simulink model "Model"  (R2020a)
settings: Solver=ode4  StartTime=0.0  StopTime=100  FixedStep=0.0005  RelTol=1e-3  EnableMultiTasking=on
libraries: simulink x2
settings Model: Creator=Cason  LastModifiedBy=Cason
settings OptimizationCC: BlockReduction=off  DefaultParameterBehavior=Inlined  BufferReuse=off

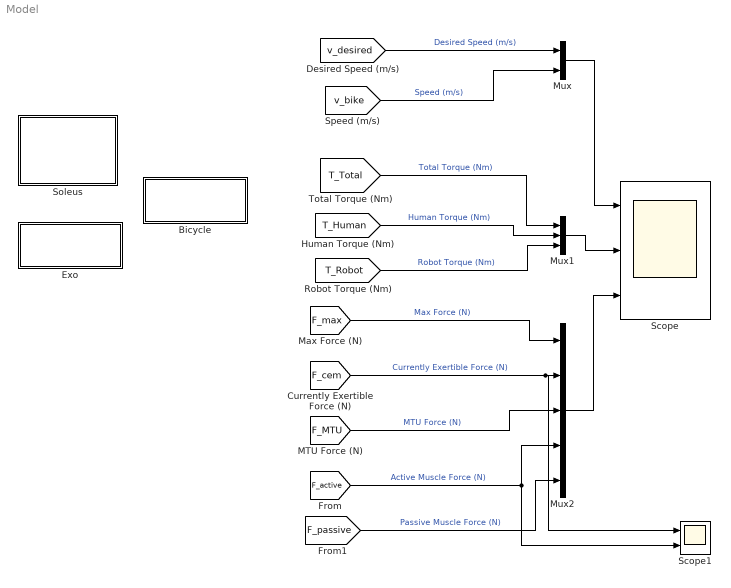
== system Model ==
  Bicycle : Subsystem
  Exo : Subsystem
  Mux : Mux  Inputs=2
  Mux1 : Mux  Inputs=3
  Mux2 : Mux  Inputs=5
  Scope : Scope  NumInputPorts=3
  Scope1 : Scope  NumInputPorts=2
  Soleus : Subsystem
  wires:
  Mux/1 -> Scope/1
  [v_desired] -> Mux/1  "Desired Speed (m/s)"
  [v_bike] -> Mux/2  "Speed (m/s)"
  Mux1/1 -> Scope/2
  [T_Human] -> Mux1/2  "Human Torque (Nm)"
  [T_Robot] -> Mux1/3  "Robot Torque (Nm)"
  [T_Total] -> Mux1/1  "Total Torque (Nm)"
  [F_max] -> Mux2/1  "Max Force (N)"
  [F_cem] -> Scope1/1, Mux2/2  "Currently Exertible Force (N)"
  [F_MTU] -> Mux2/3  "MTU Force (N)"
  Mux2/1 -> Scope/3
  [F_active] -> Scope1/2, Mux2/4  "Active Muscle Force (N)"
  [F_passive] -> Mux2/5  "Passive Muscle Force (N)"

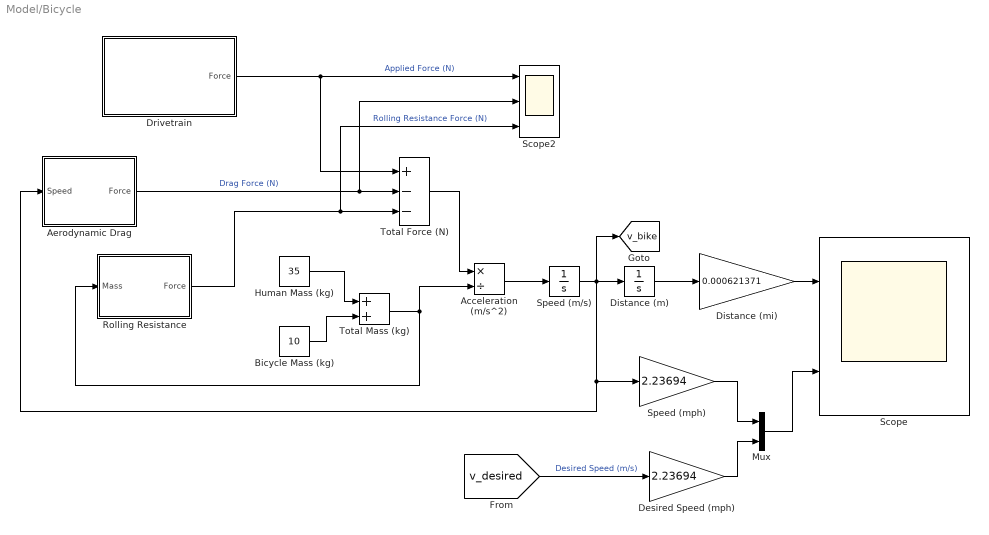
== system Model/Bicycle ==
  Acceleration (m/s^2) : Product  Inputs=*/
  Aerodynamic Drag : Subsystem
  Bicycle Mass (kg) : Constant  Value=10
  Desired Speed (mph) : Gain  Gain=2.23694
  Distance (m) : Integrator
  Distance (mi) : Gain  Gain=0.000621371
  Drivetrain : Subsystem
  Human Mass (kg) : Constant  Value=35
  Mux : Mux  Inputs=2
  Rolling Resistance : Subsystem
  Scope : Scope  NumInputPorts=2
  Scope2 : Scope  NumInputPorts=3
  Speed (m/s) : Integrator
  Speed (mph) : Gain  Gain=2.23694
  Total Force (N) : Sum  Inputs=+--
  Total Mass (kg) : Sum
  tag scope: v_bike=global
  wires:
  Human Mass (kg)/1 -> Total Mass (kg)/1
  Bicycle Mass (kg)/1 -> Total Mass (kg)/2
  Total Mass (kg)/1 -> Acceleration (m/s^2)/2, Rolling Resistance/1(Mass)
  Acceleration (m/s^2)/1 -> Speed (m/s)/1
  Speed (m/s)/1 -> [v_bike], Aerodynamic Drag/1(Speed), Speed (mph)/1, Distance (m)/1
  Distance (m)/1 -> Distance (mi)/1
  Total Force (N)/1 -> Acceleration (m/s^2)/1
  Rolling Resistance/1(Force) -> Total Force (N)/3, Scope2/3  "Rolling Resistance Force (N)"
  Aerodynamic Drag/1(Force) -> Scope2/2, Total Force (N)/2  "Drag Force (N)"
  Drivetrain/1(Force) -> Scope2/1, Total Force (N)/1  "Applied Force (N)"
  Distance (mi)/1 -> Scope/1
  Speed (mph)/1 -> Mux/1
  Mux/1 -> Scope/2
  [v_desired] -> Desired Speed (mph)/1  "Desired Speed (m/s)"
  Desired Speed (mph)/1 -> Mux/2

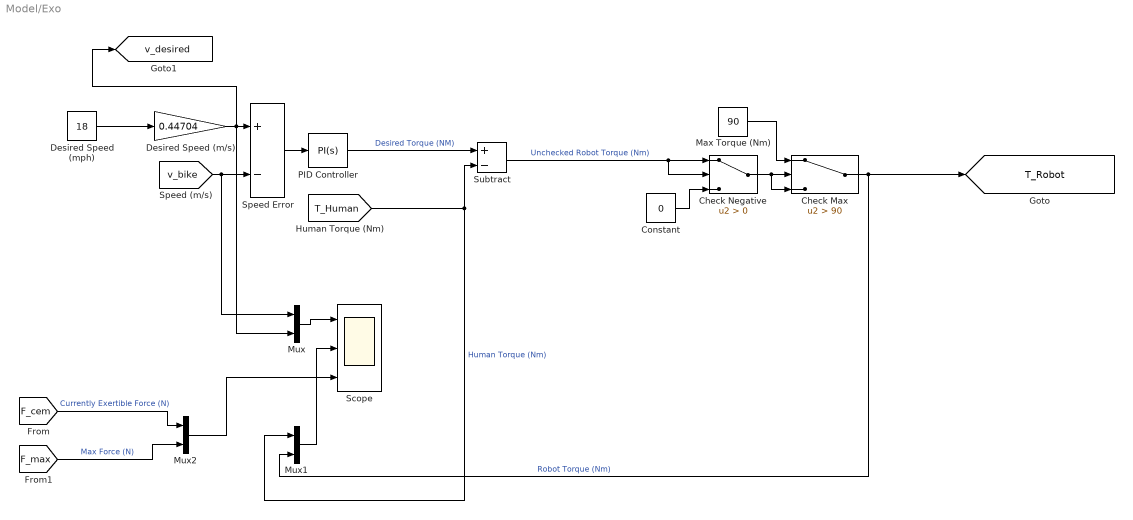
== system Model/Exo ==
  Check Max : Switch  Criteria=u2 > Threshold  Threshold=90
  Check Negative : Switch  Criteria=u2 > Threshold
  Constant : Constant  Value=0
  Desired Speed (m/s) : Gain  Gain=0.44704
  Desired Speed (mph) : Constant  Value=18
  Max Torque (Nm) : Constant  Value=90
  Mux : Mux  Inputs=2
  Mux1 : Mux  Inputs=2
  Mux2 : Mux  Inputs=2
  PID Controller : simulink/Continuous/PID Controller  Controller=PI  Form=Parallel  TimeDomain=Continuous-time  UseExternalTs=off  SampleTime=-1  IntegratorMethod=Forward Euler  FilterMethod=Forward Euler  ControllerParametersSource=internal  P=5  I=0.9  D=0.1  UseFilter=on  N=100  TunerSelectOption=Transfer Function Based (PID Tuner App)  InitialConditionSource=internal  InitialConditionForIntegrator=0  InitialConditionForFilter=0  DifferentiatorICPrevScaledInput=0  ExternalReset=none  TrackingMode=off  Kt=1  LimitOutput=off  UpperSaturationLimit=inf  LowerSaturationLimit=-inf  LinearizeAsGain=on  AntiWindupMode=none  Kb=1  POutMin=[]  POutMax=[]  IOutMin=[]  IOutMax=[]  DOutMin=[]  DOutMax=[]  NOutMin=[]  NOutMax=[]  SumOutMin=[]  SumOutMax=[]  SaturationOutMin=[]  SaturationOutMax=[]  PParamMin=[]  PParamMax=[]  IParamMin=[]  IParamMax=[]  DParamMin=[]  DParamMax=[]  NParamMin=[]  NParamMax=[]  KbParamMin=[]  KbParamMax=[]  KtParamMin=[]  KtParamMax=[]  KbOutMin=[]  KbOutMax=[]  KtOutMin=[]  KtOutMax=[]  IntegratorOutMin=[]  IntegratorOutMax=[]  FilterOutMin=[]  FilterOutMax=[]  SumI1OutMin=[]  SumI1OutMax=[]  SumI2OutMin=[]  SumI2OutMax=[]  SumI3OutMin=[]  SumI3OutMax=[]  SumI4OutMin=[]  SumI4OutMax=[]  SumDOutMin=[]  SumDOutMax=[]  DifferentiatorOutMin=[]  DifferentiatorOutMax=[]  FilterDiffOutCoefMin=[]  FilterDiffOutCoefMax=[]  ReciprocalOutMin=[]  ReciprocalOutMax=[]  SumDenOutMin=[]  SumDenOutMax=[]  SumNumOutMin=[]  SumNumOutMax=[]  DivideOutMin=[]  DivideOutMax=[]  UdiffTsProdOutMin=[]  UdiffTsProdOutMax=[]  NTsProdOutMin=[]  NTsProdOutMax=[]  UintegralTsProdOutMin=[]  UintegralTsProdOutMax=[]  UngainTsProdOutMin=[]  UngainTsProdOutMax=[]  IntegratorContinuousStateAttributes=''  IntegratorStateMustResolveToSignalObject=off  IntegratorRTWStateStorageClass=Auto  FilterContinuousStateAttributes=''  FilterStateMustResolveToSignalObject=off  FilterRTWStateStorageClass=Auto  ParallelPVariant=InternalParameters  IdealPVariant=Disabled  IVariant=InternalParameters  DVariant=Disabled  IntegratorVariant=Continuous  SatVariant=Disabled  AWVariant=Passthrough  PCopyVariant=Disabled  TRVariant=Disabled  FdbkBlocksVariant=Forward  IdealPFdbkVariant=Disabled  SatFdbkVariant=Disabled  DerivativeFilterVariant=Disabled  NVariant=Disabled  NCopyVariant=Disabled_SignalSpec  FilterICVariant=Disabled  IntegratorICVariant=InternalICs  ExternalResetVariant=Disabled  TRSumVariant=Passthrough  SumFdbkVariant=Disabled  SumVariant=Sum_PI  TsampFilterVariant=InternalTs  TsampNgainVariant=Passthrough  TsampIntegralVariant=Passthrough
  Scope : Scope  NumInputPorts=3
  Speed Error : Sum  Inputs=+-
  Subtract : Sum  Inputs=+-
  tag scope: T_Robot=global, v_desired=global
  wires:
  Desired Speed (mph)/1 -> Desired Speed (m/s)/1
  Desired Speed (m/s)/1 -> [v_desired], Mux/2, Speed Error/1
  [v_bike] -> Mux/1, Speed Error/2
  Speed Error/1 -> PID Controller/1
  PID Controller/1 -> Subtract/1  "Desired Torque (NM)"
  Subtract/1 -> Check Negative/2, Check Negative/1  "Unchecked Robot Torque (Nm)"
  [T_Human] -> Mux1/1, Subtract/2  "Human Torque (Nm)"
  Constant/1 -> Check Negative/3
  Check Negative/1 -> Check Max/3, Check Max/2
  Max Torque (Nm)/1 -> Check Max/1
  Check Max/1 -> [T_Robot], Mux1/2  "Robot Torque (Nm)"
  Mux/1 -> Scope/1
  Mux1/1 -> Scope/2
  Mux2/1 -> Scope/3
  [F_cem] -> Mux2/1  "Currently Exertible Force (N)"
  [F_max] -> Mux2/2  "Max Force (N)"

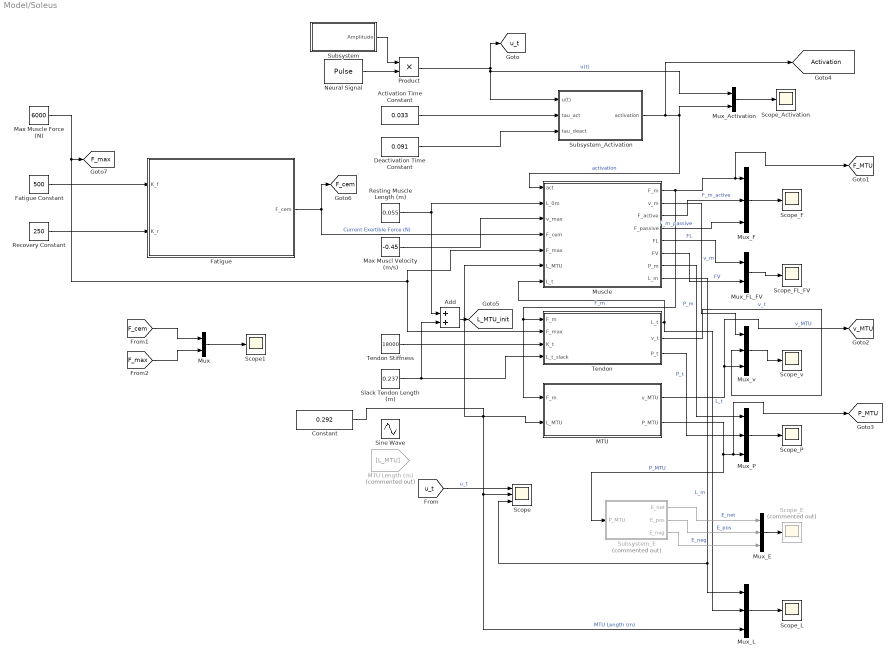
== system Model/Soleus ==
  Activation Time Constant : Constant  Value=0.033
  Add : Sum
  Constant : Constant  Value=0.292
  Deactivation Time Constant : Constant  Value=0.091
  Fatigue : Subsystem
  Fatigue Constant : Constant  Value=500
  MTU : Subsystem
  MTU Length (m) : From  Commented=on  GotoTag=L_MTU
  Max Muscl Velocity (m/s) : Constant  Value=-0.45
  Max Muscle Force (N) : Constant  Value=6000
  Muscle : Subsystem
  Mux : Mux  Inputs=2
  Mux_Activation : Mux  Inputs=2
  Mux_E : Mux  Inputs=3
  Mux_F : Mux  Inputs=3
  Mux_FL_FV : Mux  Inputs=2
  Mux_L : Mux  Inputs=3
  Mux_P : Mux  Inputs=3
  Mux_v : Mux  Inputs=3
  Neural Signal : DiscretePulseGenerator  PulseType=Time based  Period=0.75  PulseWidth=50
  Product : Product
  Recovery Constant : Constant  Value=250
  Resting Muscle Length (m) : Constant  Value=0.055
  Scope : Scope  NumInputPorts=3
  Scope1 : Scope
  Scope_Activation : Scope
  Scope_E : Scope  Commented=on
  Scope_F : Scope
  Scope_FL_FV : Scope
  Scope_L : Scope
  Scope_P : Scope
  Scope_v : Scope
  Sine Wave : Sin  Amplitude=0.05*0.292  Bias=0.292  Frequency=2.66*pi  Phase=pi/2  SampleTime=0
  Slack Tendon Length (m) : Constant  Value=0.237
  Subsystem : Subsystem
  Subsystem_Activation : Subsystem
  Subsystem_E : Subsystem  Commented=on
  Tendon : Subsystem
  Tendon Stiffness : Constant  Value=18000
  tag scope: Activation=global, F_MTU=global, F_cem=global, F_max=global, L_MTU_init=global, P_MTU=global, u_t=global, v_MTU=global
  wires:
  Mux_v/1 -> Scope_v/1
  Product/1 -> [u_t], Mux_Activation/1, Subsystem_Activation/1(u(t))  "u(t)"
  Muscle/7(P_m) -> Mux_P/1  "P_m"
  Activation Time Constant/1 -> Subsystem_Activation/2(tau_act)
  Tendon Stiffness/1 -> Tendon/3(K_t)
  Mux_F/1 -> Scope_F/1
  MTU/2(P_MTU) -> Subsystem_E/1(P_MTU), [P_MTU], Mux_P/3  "P_MTU"
  Tendon/2(v_t) -> Mux_v/2  "v_t"
  Slack Tendon Length (m)/1 -> Add/2, Tendon/4(L_t_slack)
  Mux_P/1 -> Scope_P/1
  Tendon/1(L_t) -> Mux_L/2, Muscle/7(L_t)  "L_t"
  Mux_Activation/1 -> Scope_Activation/1
  MTU/1(v_MTU) -> [v_MTU], Mux_v/3  "v_MTU"
  Muscle/8(L_m) -> Mux_L/1, Scope/3  "L_m"
  Muscle/5(FL) -> Mux_FL_FV/1  "FL"
  Max Muscl Velocity (m/s)/1 -> Muscle/3(v_max)
  Resting Muscle Length (m)/1 -> Muscle/2(L_0m), Add/1
  Muscle/6(FV) -> Mux_FL_FV/2  "FV"
  Tendon/3(P_t) -> Mux_P/2  "P_t"
  Muscle/4(F_passive) -> Mux_F/3  "F_m_passive"
  Muscle/2(v_m) -> Mux_v/1  "v_m"
  Deactivation Time Constant/1 -> Subsystem_Activation/3(tau_deact)
  Mux_FL_FV/1 -> Scope_FL_FV/1
  Muscle/3(F_active) -> Mux_F/2  "F_m_active"
  Subsystem_Activation/1(activation) -> [Activation], Mux_Activation/2, Muscle/1(act)  "activation"
  Mux_L/1 -> Scope_L/1
  Muscle/1(F_m) -> MTU/1(F_m), Tendon/1(F_m), [F_MTU], Mux_F/1  "F_m"
  Mux_E/1 -> Scope_E/1
  Subsystem_E/1(E_net) -> Mux_E/1  "E_net"
  Subsystem_E/2(E_pos) -> Mux_E/2  "E_pos"
  Subsystem_E/3(E_neg) -> Mux_E/3  "E_neg"
  Constant/1 -> Mux_L/3, Scope/2, Muscle/6(L_MTU), MTU/2(L_MTU)  "MTU Length (m)"
  [u_t] -> Scope/1  "u_t"
  Add/1 -> [L_MTU_init]
  Max Muscle Force (N)/1 -> Muscle/5(F_max), Tendon/2(F_max), [F_max]
  Fatigue Constant/1 -> Fatigue/1(K_f)
  Recovery Constant/1 -> Fatigue/2(K_r)
  Mux/1 -> Scope1/1
  [F_cem] -> Mux/1
  [F_max] -> Mux/2
  Fatigue/1(F_cem) -> [F_cem], Muscle/4(F_cem)  "Current Exertible Force (N)"
  Neural Signal/1 -> Product/2
  Subsystem/1(Amplitude) -> Product/1

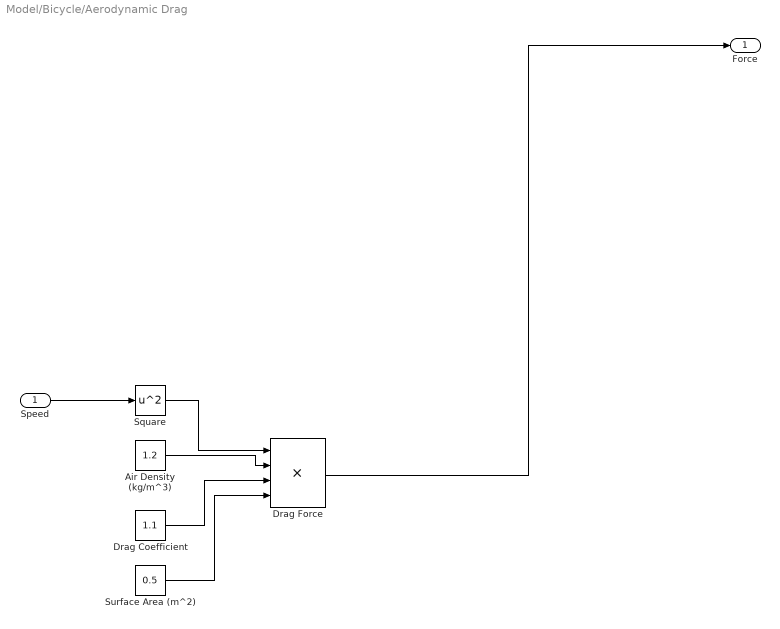
== system Model/Bicycle/Aerodynamic Drag ==
  Speed : Inport
  Air Density (kg/m^3) : Constant  Value=1.2
  Drag Coefficient : Constant  Value=1.1
  Drag Force : Product  Inputs=4
  Square : Math  Operator=square  SaturateOnIntegerOverflow=on
  Surface Area (m^2) : Constant  Value=0.5
  Force : Outport
  wires:
  Air Density (kg/m^3)/1 -> Drag Force/2
  Drag Coefficient/1 -> Drag Force/3
  Square/1 -> Drag Force/1
  Drag Force/1 -> Force/1
  Surface Area (m^2)/1 -> Drag Force/4
  Speed/1 -> Square/1

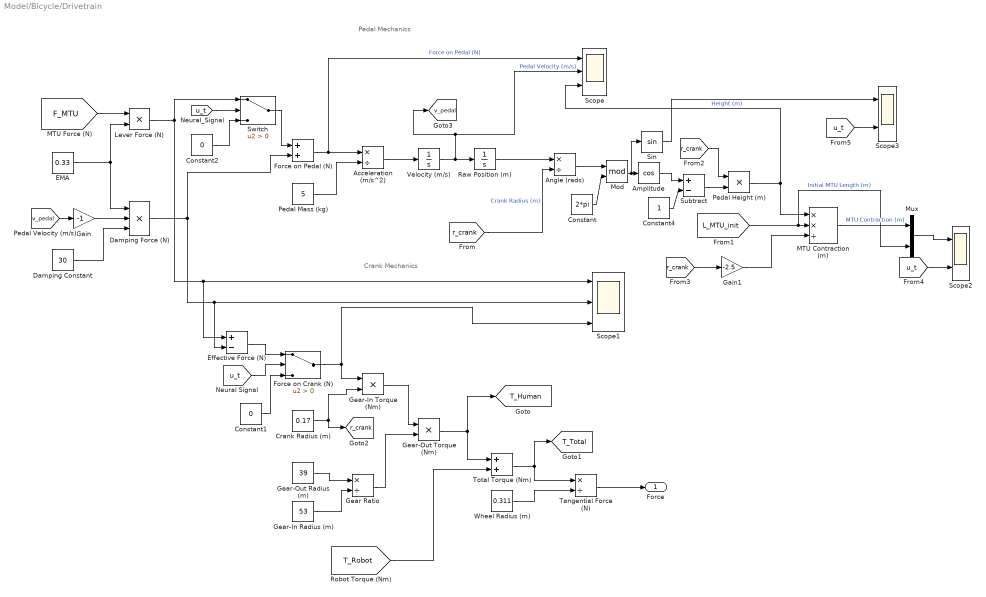
== system Model/Bicycle/Drivetrain ==
  note: Pedal Mechanics
  note: Crank Mechanics
  Acceleration (m/s^2) : Product  Inputs=*/
  Amplitude : Trigonometry  Operator=cos
  Angle (rads) : Product  Inputs=*/
  Constant : Constant  Value=2*pi
  Constant1 : Constant  Value=0
  Constant2 : Constant  Value=0
  Constant4 : Constant
  Crank Radius (m) : Constant  Value=0.17
  Damping Constant : Constant  Value=30
  Damping Force (N) : Product  Inputs=3
  EMA : Constant  Value=0.33
  Effective Force (N) : Sum  Inputs=+-
  Force on Crank (N) : Switch  Criteria=u2 > Threshold
  Force on Pedal (N) : Sum
  Gain : Gain  Gain=-1
  Gain1 : Gain  Gain=-2.5
  Gear Ratio : Product  Inputs=*/
  Gear-In Radius (m) : Constant  Value=53
  Gear-In Torque (Nm) : Product
  Gear-Out Radius (m) : Constant  Value=39
  Gear-Out Torque (Nm) : Product
  Lever Force (N) : Product
  MTU Contraction (m) : Product  Inputs=**/
  Mod : Math  Operator=mod  SaturateOnIntegerOverflow=on
  Mux : Mux  Inputs=2
  Pedal Height (m) : Product
  Pedal Mass (kg) : Constant  Value=5
  Raw Position (m) : Integrator
  Scope : Scope  NumInputPorts=3
  Scope1 : Scope  NumInputPorts=3
  Scope2 : Scope  NumInputPorts=2
  Scope3 : Scope  NumInputPorts=2
  Sin : Trigonometry
  Subtract : Sum  Inputs=+-
  Switch : Switch  Criteria=u2 > Threshold
  Tangential Force (N) : Product  Inputs=*/
  Total Torque (Nm) : Sum
  Velocity (m/s) : Integrator
  Wheel Radius (m) : Constant  Value=0.311
  Force : Outport
  tag scope: T_Human=global, T_Total=global, r_crank=global, v_pedal=global
  wires:
  Gear-In Radius (m)/1 -> Gear Ratio/2
  Gear-In Torque (Nm)/1 -> Gear-Out Torque (Nm)/1
  Total Torque (Nm)/1 -> [T_Total], Tangential Force (N)/1
  EMA/1 -> Lever Force (N)/2, Damping Force (N)/1
  Damping Constant/1 -> Damping Force (N)/3
  Lever Force (N)/1 -> Switch/1, Effective Force (N)/1, Scope1/1
  Gear-Out Torque (Nm)/1 -> [T_Human], Total Torque (Nm)/1
  Damping Force (N)/1 -> Force on Pedal (N)/2, Effective Force (N)/2, Scope1/2
  Gear-Out Radius (m)/1 -> Gear Ratio/1
  Gain/1 -> Damping Force (N)/2
  Gear Ratio/1 -> Gear-Out Torque (Nm)/2
  Effective Force (N)/1 -> Force on Crank (N)/1
  [F_MTU] -> Lever Force (N)/1
  Force on Crank (N)/1 -> Scope1/3, Gear-In Torque (Nm)/1
  Crank Radius (m)/1 -> [r_crank], Gear-In Torque (Nm)/2
  [u_t] -> Force on Crank (N)/2
  Constant1/1 -> Force on Crank (N)/3
  Wheel Radius (m)/1 -> Tangential Force (N)/2
  [v_pedal] -> Gain/1
  Tangential Force (N)/1 -> Force/1
  [T_Robot] -> Total Torque (Nm)/2
  [u_t] -> Switch/2
  Constant2/1 -> Switch/3
  Switch/1 -> Force on Pedal (N)/1
  Force on Pedal (N)/1 -> Scope/1, Acceleration (m/s^2)/1  "Force on Pedal (N)"
  Pedal Mass (kg)/1 -> Acceleration (m/s^2)/2
  Acceleration (m/s^2)/1 -> Velocity (m/s)/1
  Velocity (m/s)/1 -> Raw Position (m)/1, Scope/2, [v_pedal]  "Pedal Velocity (m/s)"
  Raw Position (m)/1 -> Angle (rads)/1
  [r_crank] -> Angle (rads)/2  "Crank Radius (m)"
  Constant/1 -> Mod/2
  Angle (rads)/1 -> Mod/1
  Mod/1 -> Sin/1, Amplitude/1
  Pedal Height (m)/1 -> MTU Contraction (m)/1, Scope/3  "Height (m)"
  Gain1/1 -> MTU Contraction (m)/3
  [L_MTU_init] -> Mux/2, MTU Contraction (m)/2  "Initial MTU Length (m)"
  MTU Contraction (m)/1 -> Mux/1  "MTU Contraction (m)"
  Constant4/1 -> Subtract/2
  Amplitude/1 -> Subtract/1
  Subtract/1 -> Pedal Height (m)/2
  [r_crank] -> Pedal Height (m)/1
  [r_crank] -> Gain1/1
  Mux/1 -> Scope2/1
  [u_t] -> Scope2/2
  [u_t] -> Scope3/2
  Sin/1 -> Scope3/1

== system Model/Bicycle/Rolling Resistance ==
  Mass : Inport
  Friction Force (N) : Product
  Gravitational Force (N) : Product
  Gravity (m/s^2) : Constant  Value=9.81
  Rolling Resistance Coefficient : Constant  Value=0.002
  Force : Outport
  wires:
  Mass/1 -> Gravitational Force (N)/2
  Rolling Resistance Coefficient/1 -> Friction Force (N)/1
  Gravity (m/s^2)/1 -> Gravitational Force (N)/1
  Friction Force (N)/1 -> Force/1
  Gravitational Force (N)/1 -> Friction Force (N)/2

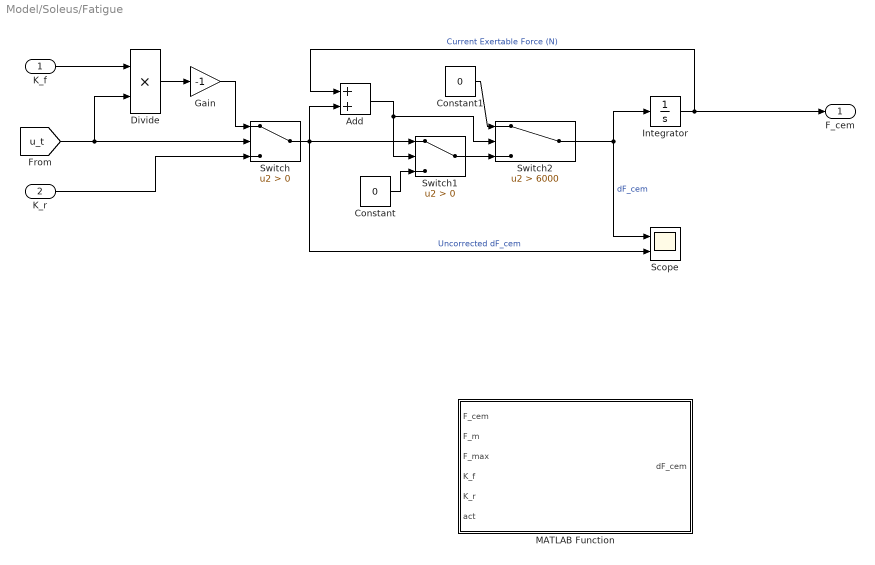
== system Model/Soleus/Fatigue ==
  K_f : Inport
  K_r : Inport  Port=2
  Add : Sum
  Constant : Constant  Value=0
  Constant1 : Constant  Value=0
  Divide : Product  Inputs=**
  Gain : Gain  Gain=-1
  Integrator : Integrator  InitialCondition=6000
  MATLAB Function : MATLAB Function  TreatAsAtomicUnit=on
  Scope : Scope  NumInputPorts=2
  Switch : Switch  Criteria=u2 > Threshold
  Switch1 : Switch  Criteria=u2 > Threshold
  Switch2 : Switch  Criteria=u2 > Threshold  Threshold=6000
  F_cem : Outport
  wires:
  Switch2/1 -> Scope/1, Integrator/1  "dF_cem"
  Integrator/1 -> Add/1, F_cem/1  "Current Exertable Force (N)"
  K_f/1 -> Divide/1
  [u_t] -> Switch/2, Divide/2
  Divide/1 -> Gain/1
  K_r/1 -> Switch/3
  Gain/1 -> Switch/1
  Switch/1 -> Scope/2, Switch1/1, Add/2  "Uncorrected dF_cem"
  Add/1 -> Switch1/2, Switch2/2
  Constant/1 -> Switch1/3
  Switch1/1 -> Switch2/3
  Constant1/1 -> Switch2/1

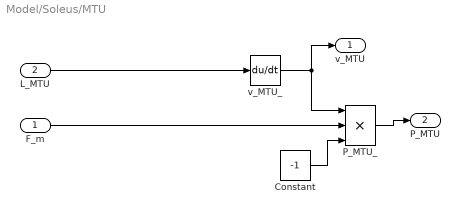
== system Model/Soleus/MTU ==
  F_m : Inport
  L_MTU : Inport  Port=2
  Constant : Constant  Value=-1
  P_MTU_ : Product  Inputs=3
  v_MTU_ : Derivative
  v_MTU : Outport
  P_MTU : Outport  Port=2
  wires:
  v_MTU_/1 -> P_MTU_/1, v_MTU/1
  F_m/1 -> P_MTU_/2
  P_MTU_/1 -> P_MTU/1
  Constant/1 -> P_MTU_/3
  L_MTU/1 -> v_MTU_/1

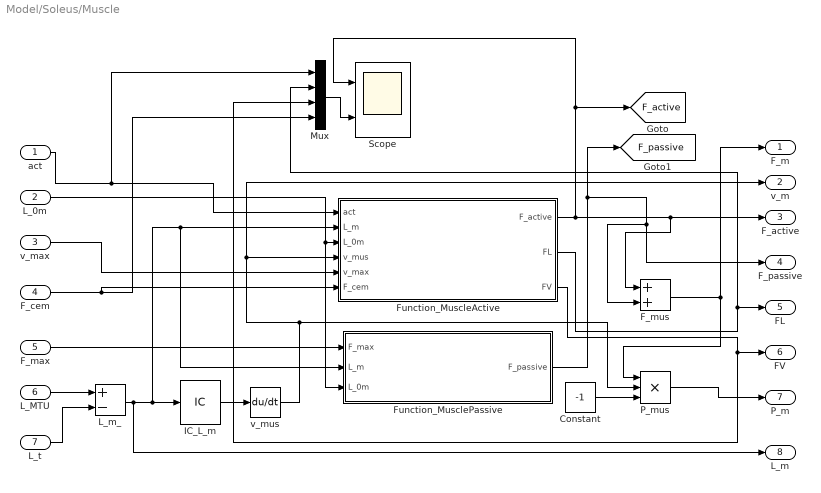
== system Model/Soleus/Muscle ==
  act : Inport
  L_0m : Inport  Port=2
  v_max : Inport  Port=3
  F_cem : Inport  Port=4
  F_max : Inport  Port=5
  L_MTU : Inport  Port=6
  L_t : Inport  Port=7
  Constant : Constant  Value=-1
  F_mus : Sum
  Function_MuscleActive : MATLAB Function  TreatAsAtomicUnit=on
  Function_MusclePassive : MATLAB Function  TreatAsAtomicUnit=on
  IC_L_m : InitialCondition  Value=0.055
  L_m_ : Sum  Inputs=+-
  Mux : Mux
  P_mus : Product  Inputs=3
  Scope : Scope  NumInputPorts=2
  v_mus : Derivative
  F_m : Outport
  v_m : Outport  Port=2
  F_active : Outport  Port=3
  F_passive : Outport  Port=4
  FL : Outport  Port=5
  FV : Outport  Port=6
  P_m : Outport  Port=7
  L_m : Outport  Port=8
  tag scope: F_active=global, F_passive=global
  wires:
  L_t/1 -> L_m_/2
  IC_L_m/1 -> v_mus/1
  Function_MusclePassive/1(F_passive) -> [F_passive], F_passive/1, F_mus/2
  L_m_/1 -> L_m/1, IC_L_m/1, Function_MuscleActive/2(L_m), Function_MusclePassive/2(L_m)
  L_0m/1 -> Function_MusclePassive/3(L_0m), Function_MuscleActive/3(L_0m)
  v_mus/1 -> v_m/1, Function_MuscleActive/4(v_mus), P_mus/2
  Function_MuscleActive/2(FL) -> Mux/2, FL/1
  Function_MuscleActive/1(F_active) -> Scope/1, [F_active], F_mus/1, F_active/1
  act/1 -> Mux/1, Function_MuscleActive/1(act)
  v_max/1 -> Function_MuscleActive/5(v_max)
  F_mus/1 -> F_m/1, P_mus/1
  F_max/1 -> Function_MusclePassive/1(F_max)
  P_mus/1 -> P_m/1
  Function_MuscleActive/3(FV) -> Mux/3, FV/1
  Constant/1 -> P_mus/3
  L_MTU/1 -> L_m_/1
  F_cem/1 -> Mux/4, Function_MuscleActive/6(F_cem)
  Mux/1 -> Scope/2

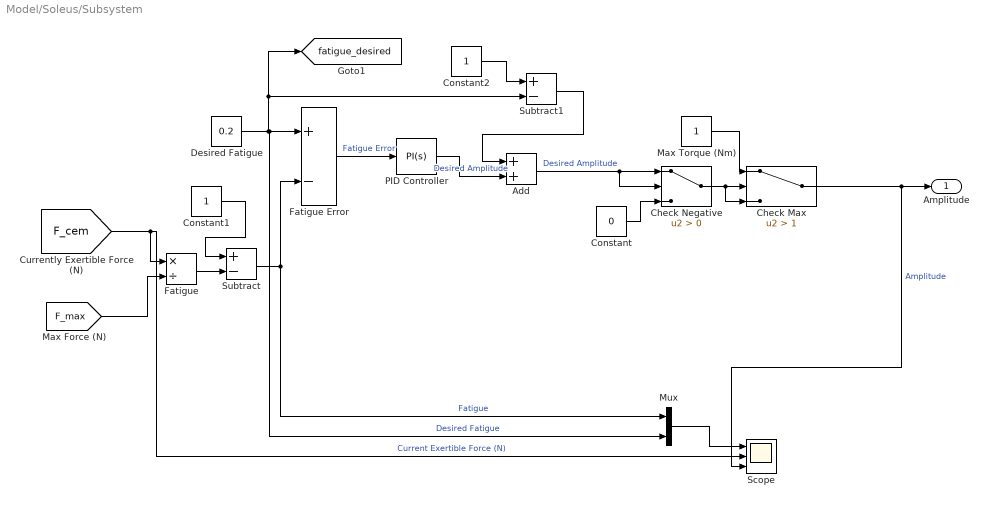
== system Model/Soleus/Subsystem ==
  Add : Sum
  Check Max : Switch  Criteria=u2 > Threshold  Threshold=1
  Check Negative : Switch  Criteria=u2 > Threshold
  Constant : Constant  Value=0
  Constant1 : Constant
  Constant2 : Constant
  Desired Fatigue : Constant  Value=0.2
  Fatigue : Product  Inputs=*/
  Fatigue Error : Sum  Inputs=+-
  Max Torque (Nm) : Constant
  Mux : Mux  Inputs=2
  PID Controller : simulink/Continuous/PID Controller  Controller=PI  Form=Parallel  TimeDomain=Continuous-time  UseExternalTs=off  SampleTime=-1  IntegratorMethod=Forward Euler  FilterMethod=Forward Euler  ControllerParametersSource=internal  P=8  I=0.6  D=0.8  UseFilter=on  N=100  TunerSelectOption=Transfer Function Based (PID Tuner App)  InitialConditionSource=internal  InitialConditionForIntegrator=0  InitialConditionForFilter=0  DifferentiatorICPrevScaledInput=0  ExternalReset=none  TrackingMode=off  Kt=1  LimitOutput=off  UpperSaturationLimit=inf  LowerSaturationLimit=-inf  LinearizeAsGain=on  AntiWindupMode=none  Kb=1  POutMin=[]  POutMax=[]  IOutMin=[]  IOutMax=[]  DOutMin=[]  DOutMax=[]  NOutMin=[]  NOutMax=[]  SumOutMin=[]  SumOutMax=[]  SaturationOutMin=[]  SaturationOutMax=[]  PParamMin=[]  PParamMax=[]  IParamMin=[]  IParamMax=[]  DParamMin=[]  DParamMax=[]  NParamMin=[]  NParamMax=[]  KbParamMin=[]  KbParamMax=[]  KtParamMin=[]  KtParamMax=[]  KbOutMin=[]  KbOutMax=[]  KtOutMin=[]  KtOutMax=[]  IntegratorOutMin=[]  IntegratorOutMax=[]  FilterOutMin=[]  FilterOutMax=[]  SumI1OutMin=[]  SumI1OutMax=[]  SumI2OutMin=[]  SumI2OutMax=[]  SumI3OutMin=[]  SumI3OutMax=[]  SumI4OutMin=[]  SumI4OutMax=[]  SumDOutMin=[]  SumDOutMax=[]  DifferentiatorOutMin=[]  DifferentiatorOutMax=[]  FilterDiffOutCoefMin=[]  FilterDiffOutCoefMax=[]  ReciprocalOutMin=[]  ReciprocalOutMax=[]  SumDenOutMin=[]  SumDenOutMax=[]  SumNumOutMin=[]  SumNumOutMax=[]  DivideOutMin=[]  DivideOutMax=[]  UdiffTsProdOutMin=[]  UdiffTsProdOutMax=[]  NTsProdOutMin=[]  NTsProdOutMax=[]  UintegralTsProdOutMin=[]  UintegralTsProdOutMax=[]  UngainTsProdOutMin=[]  UngainTsProdOutMax=[]  IntegratorContinuousStateAttributes=''  IntegratorStateMustResolveToSignalObject=off  IntegratorRTWStateStorageClass=Auto  FilterContinuousStateAttributes=''  FilterStateMustResolveToSignalObject=off  FilterRTWStateStorageClass=Auto  ParallelPVariant=InternalParameters  IdealPVariant=Disabled  IVariant=InternalParameters  DVariant=Disabled  IntegratorVariant=Continuous  SatVariant=Disabled  AWVariant=Passthrough  PCopyVariant=Disabled  TRVariant=Disabled  FdbkBlocksVariant=Forward  IdealPFdbkVariant=Disabled  SatFdbkVariant=Disabled  DerivativeFilterVariant=Disabled  NVariant=Disabled  NCopyVariant=Disabled_SignalSpec  FilterICVariant=Disabled  IntegratorICVariant=InternalICs  ExternalResetVariant=Disabled  TRSumVariant=Passthrough  SumFdbkVariant=Disabled  SumVariant=Sum_PI  TsampFilterVariant=InternalTs  TsampNgainVariant=Passthrough  TsampIntegralVariant=Passthrough
  Scope : Scope  NumInputPorts=3
  Subtract : Sum  Inputs=+-
  Subtract1 : Sum  Inputs=+-
  Amplitude : Outport
  tag scope: fatigue_desired=global
  wires:
  Check Negative/1 -> Check Max/3, Check Max/2
  Max Torque (Nm)/1 -> Check Max/1
  Check Max/1 -> Scope/3, Amplitude/1  "Amplitude"
  Constant/1 -> Check Negative/3
  Subtract/1 -> Mux/1, Fatigue Error/2  "Fatigue"
  Desired Fatigue/1 -> Mux/2, Fatigue Error/1, [fatigue_desired], Subtract1/2  "Desired Fatigue"
  Fatigue Error/1 -> PID Controller/1  "Fatigue Error"
  Add/1 -> Check Negative/2, Check Negative/1  "Desired Amplitude"
  [F_cem] -> Scope/2, Fatigue/1  "Current Exertible Force (N)"
  [F_max] -> Fatigue/2
  Constant1/1 -> Subtract/1
  Fatigue/1 -> Subtract/2
  Constant2/1 -> Subtract1/1
  Subtract1/1 -> Add/1
  PID Controller/1 -> Add/2  "Desired Amplitude"
  Mux/1 -> Scope/1

== system Model/Soleus/Subsystem_Activation ==
  u(t) : Inport
  tau_act : Inport  Port=2
  tau_deact : Inport  Port=3
  Function_Activation : MATLAB Function  TreatAsAtomicUnit=on
  a(t) : Integrator
  activation : Outport
  wires:
  Function_Activation/1(da) -> a(t)/1
  tau_deact/1 -> Function_Activation/4(tau_deact)
  tau_act/1 -> Function_Activation/3(tau_act)
  a(t)/1 -> Function_Activation/2(a), activation/1
  u(t)/1 -> Function_Activation/1(u)

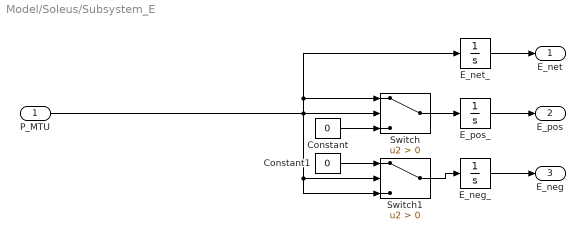
== system Model/Soleus/Subsystem_E ==
  P_MTU : Inport
  Constant : Constant  Value=0
  Constant1 : Constant  Value=0
  E_neg_ : Integrator
  E_net_ : Integrator
  E_pos_ : Integrator
  Switch : Switch  Criteria=u2 > Threshold
  Switch1 : Switch  Criteria=u2 > Threshold
  E_net : Outport
  E_pos : Outport  Port=2
  E_neg : Outport  Port=3
  wires:
  Constant/1 -> Switch/3
  E_pos_/1 -> E_pos/1
  Constant1/1 -> Switch1/1
  P_MTU/1 -> Switch1/3, Switch1/2, Switch/2, E_net_/1, Switch/1
  Switch/1 -> E_pos_/1
  Switch1/1 -> E_neg_/1
  E_neg_/1 -> E_neg/1
  E_net_/1 -> E_net/1

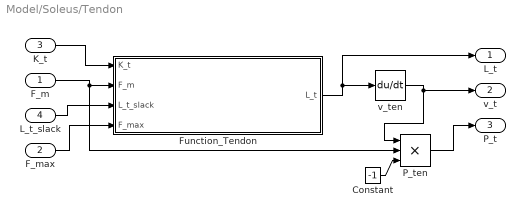
== system Model/Soleus/Tendon ==
  F_m : Inport
  F_max : Inport  Port=2
  K_t : Inport  Port=3
  L_t_slack : Inport  Port=4
  Constant : Constant  Value=-1
  Function_Tendon : MATLAB Function  TreatAsAtomicUnit=on
  P_ten : Product  Inputs=3
  v_ten : Derivative
  L_t : Outport
  v_t : Outport  Port=2
  P_t : Outport  Port=3
  wires:
  Constant/1 -> P_ten/3
  F_m/1 -> P_ten/2, Function_Tendon/2(F_m)
  L_t_slack/1 -> Function_Tendon/3(L_t_slack)
  F_max/1 -> Function_Tendon/4(F_max)
  K_t/1 -> Function_Tendon/1(K_t)
  v_ten/1 -> P_ten/1, v_t/1
  P_ten/1 -> P_t/1
  Function_Tendon/1(L_t) -> L_t/1, v_ten/1

== matlab function Model/Soleus/Muscle/Function_MuscleActive ==
  data: act input; F_active output; L_m input; L_0m input; v_mus input; v_max input; F_cem input; FL output; FV output
function [F_active, FL, FV]= active_muscle_dynamics(act, L_m, L_0m, v_mus, v_max, F_cem)
a = 3.1108; b = 0.8698; s = 0.3914;

if L_m < 0
    L_m = 0;
end

FL = exp(-abs(((L_m / L_0m)^b - 1) / s)^a);

if v_mus < v_max
    FV = 0;
elseif v_mus >= v_max && v_mus < 0  % Shortening
    FV = (1 - v_mus/v_max) / (1 + v_mus/(0.17*v_max));
else                                % Lengthening
    FV = 1.8 - 0.8*((1 + v_mus/v_max) / (1 - 7.56*(v_mus/(0.17*v_max))));
end

F_active = act * FL * FV * F_cem;

== matlab function Model/Soleus/Subsystem_Activation/Function_Activation ==
  data: u input; da output; a input; tau_act input; tau_deact input
function da = activation(u, a, tau_act, tau_deact)
beta = tau_act / tau_deact;
da = u / tau_act - (beta + (1 - beta)*u) / tau_act * a;

== matlab function Model/Soleus/Muscle/Function_MusclePassive ==
  data: F_max input; F_passive output; L_m input; L_0m input
function F_passive = passive_muscle_dynamics(F_max, L_m, L_0m)
A = 2.39E-2; b = 5.31;

F_passive = F_max*A*exp(b*(L_m/L_0m - 1));

== matlab function Model/Soleus/Tendon/Function_Tendon ==
  data: K_t input; L_t output; F_m input; L_t_slack input; F_max input
function L_t = tendon_dynamics(K_t, F_m, L_t_slack, F_max)
D_L_t = (F_m + (F_max*log(-9*exp(-(20*F_m)/F_max)+ 10)) / 20) / K_t;
L_t = D_L_t + L_t_slack;

== matlab function Model/Soleus/Fatigue/MATLAB Function ==
  data: F_cem input; dF_cem output; F_m input; F_max input; K_f input; K_r input; act input
function dF_cem = fatigue(F_cem, F_m, F_max, K_f, K_r, act)
temp = (act)*-K_f*F_cem/F_max*F_m + (1 - act)*K_r;

if F_cem + temp < 0
    dF_cem = -F_cem;
elseif F_cem + temp > F_max
    dF_cem = F_max - F_cem;
else
    dF_cem = temp;
end
